simulink model "real_system"  (R2025a)
settings: Solver=FixedStepAuto  StartTime=0.0  StopTime=inf  RelTol=1e-3
libraries: instrumentseriallib x3
settings Model: SimulationMode=accelerator  Creator=nopla  LastModifiedBy=nopla
settings OptimizationCC: UseDivisionForNetSlopeComputation=on

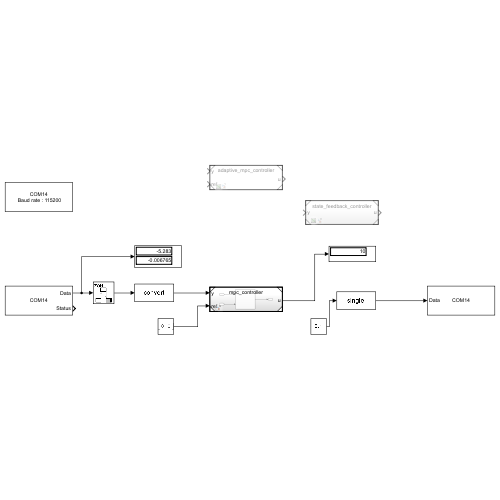
[thumbnail: Simulink's stored preview of the top-level diagram]
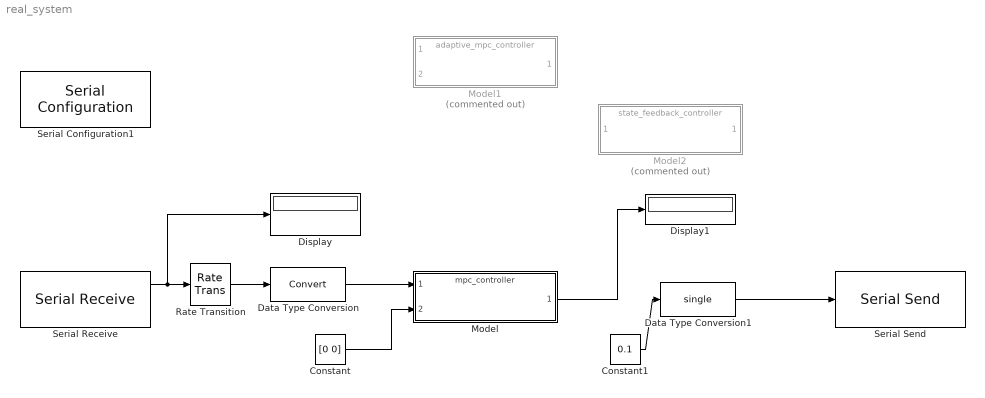
== system real_system ==
  Constant : Constant  Value=[0 0]
  Constant1 : Constant  Value=0.1  SampleTime=0.01
  Data Type Conversion : DataTypeConversion  SaturateOnIntegerOverflow=off  RndMeth=Floor
  Data Type Conversion1 : DataTypeConversion  OutDataTypeStr=single  SaturateOnIntegerOverflow=off  RndMeth=Floor
  Display : Display
  Display1 : Display
  Model : ModelReference  ModelNameDialog=mpc_controller.slx  SimulationMode=Normal  ModelReferenceVersion=1.11
  Model1 : ModelReference  Commented=on  ModelNameDialog=adaptive_mpc_controller.slx  SimulationMode=Normal  ModelReferenceVersion=1.25
  Model2 : ModelReference  Commented=on  ModelNameDialog=state_feedback_controller.slx  SimulationMode=Normal  ModelReferenceVersion=1.198
  Rate Transition : RateTransition
  Serial Configuration1 : instrumentseriallib/Serial Configuration  Priority=-200000  PortSel=COM14  Port=COM14  ComPort=COM14  BaudRate=115200  DataBits=8  Parity=none  StopBits=1  ByteOrder=little-endian  FlowControl=none  Timeout=1  SimulateUsing=Interpreted execution  BlockInModel=on  aMode=1
  Serial Receive : instrumentseriallib/Serial Receive  Priority=1  PortSel=COM14  Port=COM14  ComPort=COM14  DataType=single  SaveDataType=uint8  ToggleHeader=on  Header=[0x90 0x86]  ToggleDataSize=on  DataSize=[2 1]  ToggleTerminator=off  Terminator=<none>  CustomTerminator=[]  InputFormat=Column major  EnableBlockingMode=off  ActionDataUnavailable=Output last received value  ActionWhenDataUnavailable=Output last received value  CustomValue=0  SampleTime=0.001  SimulateUsing=Interpreted execution  BlockInModel=on  aMode=1  LibraryInUse=instrumentlib
  Serial Send : instrumentseriallib/Serial Send  Priority=1  PortSel=COM14  Port=COM14  ComPort=COM14  Header=[]  Terminator=<none>  CustomTerminator=[]  EnableBlockingMode=off  SimulateUsing=Interpreted execution  BlockInModel=on  aMode=1
  wires:
  Constant/1 -> Model/2
  Serial Receive/1 -> Display/1, Rate Transition/1
  Rate Transition/1 -> Data Type Conversion/1
  Data Type Conversion/1 -> Model/1
  Model/1 -> Display1/1
  Data Type Conversion1/1 -> Serial Send/1
  Constant1/1 -> Data Type Conversion1/1
